simulink subsystem "SCIRXMotorSwapHost"  (R2024b)
settings: Solver=VariableStepAuto  StartTime=0.0  StopTime=10.0  RelTol=1e-3
undefined symbols (not defined in the file or in its folder): inverter
settings Model: Creator=The MathWorks, Inc.  LastModifiedBy=snarayan
settings RTWCC: GPUComputeCapability=3.5

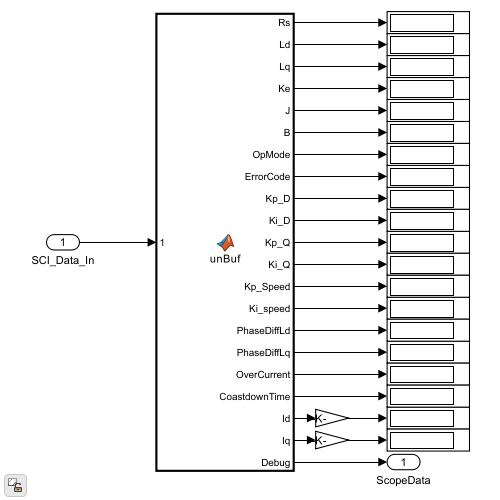
[thumbnail: Simulink's stored preview of the top-level diagram]
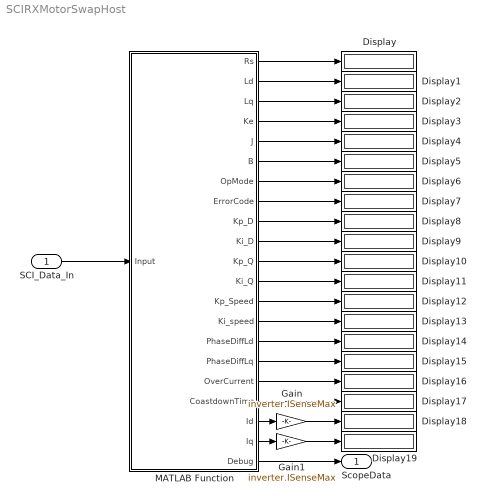
== system SCIRXMotorSwapHost ==
  SCI_Data_In : Inport
  Display{,1..19} (20 alike) : Display
  Gain : Gain  Gain=inverter.ISenseMax  OutDataTypeStr=Inherit: Same as input
  Gain1 : Gain  Gain=inverter.ISenseMax  OutDataTypeStr=Inherit: Same as input
  MATLAB Function : MATLAB Function  TreatAsAtomicUnit=on
  ScopeData : Outport
  wires:
  MATLAB Function/6(B) -> Display5/1
  MATLAB Function/7(OpMode) -> Display6/1
  MATLAB Function/8(ErrorCode) -> Display7/1
  MATLAB Function/3(Lq) -> Display2/1
  MATLAB Function/2(Ld) -> Display1/1
  MATLAB Function/1(Rs) -> Display/1
  MATLAB Function/5(J) -> Display4/1
  SCI_Data_In/1 -> MATLAB Function/1(Input)
  MATLAB Function/4(Ke) -> Display3/1
  MATLAB Function/21(Debug) -> ScopeData/1
  MATLAB Function/9(Kp_D) -> Display8/1
  MATLAB Function/10(Ki_D) -> Display9/1
  MATLAB Function/11(Kp_Q) -> Display10/1
  MATLAB Function/12(Ki_Q) -> Display11/1
  MATLAB Function/13(Kp_Speed) -> Display12/1
  MATLAB Function/14(Ki_speed) -> Display13/1
  MATLAB Function/15(PhaseDiffLd) -> Display14/1
  MATLAB Function/16(PhaseDiffLq) -> Display15/1
  MATLAB Function/17(OverCurrent) -> Display16/1
  MATLAB Function/18(CoastdownTime) -> Display17/1
  MATLAB Function/19(Id) -> Gain/1
  MATLAB Function/20(Iq) -> Gain1/1
  Gain/1 -> Display18/1
  Gain1/1 -> Display19/1

== matlab function SCIRXMotorSwapHost/MATLAB Function ==
  data: Rs output; Ld output; Lq output; Ke output; J output; B output; OpMode output; ErrorCode output; Kp_D output; Ki_D output; Kp_Q output; Ki_Q output; Kp_Speed output; Ki_speed output; PhaseDiffLd output; PhaseDiffLq output; OverCurrent output; CoastdownTime output; Id output; Iq output; Debug output; Input input
function [Rs, Ld,  Lq, Ke, J, B, OpMode, ErrorCode, Kp_D, Ki_D, Kp_Q, Ki_Q, Kp_Speed, Ki_speed, PhaseDiffLd, PhaseDiffLq, OverCurrent, CoastdownTime, Id, Iq, Debug] = unBuf(Input) 

coder.extrinsic('message', 'msgbox', 'set_param', 'error');

Rs          = Input(1, 1);
Ld          = Input(2, 1);
Lq          = Input(3, 1);
Ke          = Input(4, 1);
J           = Input(5, 1);
B           = Input(6, 1);
OpMode      = Input(7, 1);
ErrorCode   = Input(8, 1);
Kp_D        = Input(9, 1);
Ki_D        = Input(10, 1);
Kp_Q        = Input(11, 1);
Ki_Q        = Input(12, 1);
Kp_Speed    = Input(13, 1);
Ki_speed    = Input(14, 1);
PhaseDiffLd = Input(15, 1) * 180/pi;
PhaseDiffLq = Input(16, 1) * 180/pi;
OverCurrent = Input(17, 1);
CoastdownTime = Input(18, 1);
Id = Input(19, 1);
Iq = Input(20, 1);
if OverCurrent > 0 %|| UnderVoltage > 0
    set_param(bdroot, 'SimulationCommand','stop')
end

Debug = Input(:,2);
end
